simulink model "SSN_39busRT_Ctrl_4WT_19B"  (R2021a)
settings: Solver=ode3  StartTime=0.0  StopTime=10  FixedStep=Ts  MaxStep=1/60  RelTol=1e-2  AbsTol=1e-1
PreLoadFcn:
  | Ts=2.50e-6; ssn_ieee39_params; load('Pwf.mat');
InitFcn:
  | Ts=2.50e-6; ssn_ieee39_params; load('Pwf.mat');
values from neighbouring files (symbols this model uses):
  f = 50    [ssn_ieee39_params_ctrl.m]
  fNom = f    (= 60)    [ssn_ieee39_params_ctrl.m]
  ILR = 5.02    [ssn_ieee39_params_ctrl.m]
  IQMIN = 0.1    [ssn_ieee39_params_ctrl.m]
  ISCLIM = 1    [ssn_ieee39_params_ctrl.m]
  ITFpu = 1.10    (= 1.1)    [ssn_ieee39_params_ctrl.m]
  K = 1    [ssn_ieee39_params_ctrl.m]
  K1 = 1    [ssn_ieee39_params_ctrl.m]
  K2 = 2    [ssn_ieee39_params_ctrl.m]
  KCL = 1.04    [ssn_ieee39_params_ctrl.m]
  KFB = 0    [ssn_ieee39_params_ctrl.m]
  KFF = 1    [ssn_ieee39_params_ctrl.m]
  KFIX = 1    [ssn_ieee39_params_ctrl.m]
  KG = 1    [ssn_ieee39_params_ctrl.m]
  KIA = 59.91    [ssn_ieee39_params_ctrl.m]
  KIOEX = 0.0303    [ssn_ieee39_params_ctrl.m]
  KIUEX = 0.0303    [ssn_ieee39_params_ctrl.m]
  KIUOEX = 1    [ssn_ieee39_params_ctrl.m]
  KIUUEX = 1    [ssn_ieee39_params_ctrl.m]
  KLR = 22.47    [ssn_ieee39_params_ctrl.m]
  KM = 1    [ssn_ieee39_params_ctrl.m]
  KOEL = 0.24    [ssn_ieee39_params_ctrl.m]
  Kp = 1    [ssn_ieee39_params_ctrl.m]
  KPA = 30    [ssn_ieee39_params_ctrl.m]
  KPOEL = 1    [ssn_ieee39_params_ctrl.m]
  KPOEX = 0    [ssn_ieee39_params_ctrl.m]
  KPUEX = 0    [ssn_ieee39_params_ctrl.m]
  KSCALE = 0.319    [ssn_ieee39_params_ctrl.m]
  KUF = 0    [ssn_ieee39_params_ctrl.m]
  KUI = 0.001    [ssn_ieee39_params_ctrl.m]
  KUL = 0.24    [ssn_ieee39_params_ctrl.m]
  s = 10    [ssn_ieee39_params_ctrl.m]
  TA = 0.01    [ssn_ieee39_params_ctrl.m]
  Tadj = 0    [ssn_ieee39_params_ctrl.m]
  taps = [1 1 1.07 1.07 1.009 1.025 1 1.025 1.025 1.025]*1    [ssn_ieee39_params_ctrl.m]
  TF = 0.02    [ssn_ieee39_params_ctrl.m]
  TG = 0.024    [ssn_ieee39_params_ctrl.m]
  TINV = 0    [ssn_ieee39_params_ctrl.m]
  TIT = 0.1    [ssn_ieee39_params_ctrl.m]
  TL_10_11_len = 14    [ssn_ieee39_params_ctrl.m]
  TL_10_13_len = 14    [ssn_ieee39_params_ctrl.m]
  TL_13_14_len = 32    [ssn_ieee39_params_ctrl.m]
  TL_14_15_len = 70    [ssn_ieee39_params_ctrl.m]
  TL_15_16_len = 31.5    [ssn_ieee39_params_ctrl.m]
  TL_16_17_len = 26    [ssn_ieee39_params_ctrl.m]
  TL_16_19_len = 61    [ssn_ieee39_params_ctrl.m]
  TL_16_21_len = 46    [ssn_ieee39_params_ctrl.m]
  TL_16_24_len = 15    [ssn_ieee39_params_ctrl.m]
  TL_17_18_len = 26    [ssn_ieee39_params_ctrl.m]
  TL_17_27_len = 59    [ssn_ieee39_params_ctrl.m]
  TL_1_2_len = 134    [ssn_ieee39_params_ctrl.m]
  TL_1_39_len = 105    [ssn_ieee39_params_ctrl.m]
  TL_21_22_len = 47    [ssn_ieee39_params_ctrl.m]
  TL_22_23_len = 33    [ssn_ieee39_params_ctrl.m]
  TL_24_23_len = 88    [ssn_ieee39_params_ctrl.m]
  TL_25_26_len = 101    [ssn_ieee39_params_ctrl.m]
  TL_26_27_len = 46.5    [ssn_ieee39_params_ctrl.m]
  TL_26_28_len = 151    [ssn_ieee39_params_ctrl.m]
  TL_26_29_len = 200    [ssn_ieee39_params_ctrl.m]
  TL_28_29_len = 48    [ssn_ieee39_params_ctrl.m]
  TL_2_25_len = 28    [ssn_ieee39_params_ctrl.m]
  TL_2_2_len = 49    [ssn_ieee39_params_ctrl.m]
  TL_3_18_len = 42    [ssn_ieee39_params_ctrl.m]
  TL_3_4_len = 53    [ssn_ieee39_params_ctrl.m]
  TL_4_14_len = 33    [ssn_ieee39_params_ctrl.m]
  TL_4_5_len = 32.5    [ssn_ieee39_params_ctrl.m]
  TL_5_6_len = 14    [ssn_ieee39_params_ctrl.m]
  TL_5_8_len = 32    [ssn_ieee39_params_ctrl.m]
  TL_6_11_len = 26.5    [ssn_ieee39_params_ctrl.m]
  TL_6_7_len = 25.5    [ssn_ieee39_params_ctrl.m]
  TL_7_8_len = 15    [ssn_ieee39_params_ctrl.m]
  TL_8_9_len = 93    [ssn_ieee39_params_ctrl.m]
  TL_9_39_len = 136    [ssn_ieee39_params_ctrl.m]
  TOEL = 5.00    (= 5)    [ssn_ieee39_params_ctrl.m]
  TQREF = 0    [ssn_ieee39_params_ctrl.m]
  TQSCL = 0.012    [ssn_ieee39_params_ctrl.m]
  Ts_PMU = 1/1000    (= 0.001)    [ssn_ieee39_params_ctrl.m]
  TU1 = 0    [ssn_ieee39_params_ctrl.m]
  TU2 = 0    [ssn_ieee39_params_ctrl.m]
  TU3 = 0    [ssn_ieee39_params_ctrl.m]
  TU4 = 0    [ssn_ieee39_params_ctrl.m]
  TUL = 0    [ssn_ieee39_params_ctrl.m]
  TUP = 0.050    (= 0.05)    [ssn_ieee39_params_ctrl.m]
  TUQ = .005    (= 0.005)    [ssn_ieee39_params_ctrl.m]
  TUV = 0.2    [ssn_ieee39_params_ctrl.m]
  VAAMAX = VAMAX    (= 7.05)    [ssn_ieee39_params_ctrl.m]
  VAMAX = 7.05    [ssn_ieee39_params_ctrl.m]
  VAMIN = -6.11    [ssn_ieee39_params_ctrl.m]
  VBMAX = 999    [ssn_ieee39_params_ctrl.m]
  VF = 0    [ssn_ieee39_params_ctrl.m]
  VFB = 0    [ssn_ieee39_params_ctrl.m]
  VMMAX = 7.05    [ssn_ieee39_params_ctrl.m]
  VMMIN = -6.11    [ssn_ieee39_params_ctrl.m]
  VOELmax1 = 0.2353    [ssn_ieee39_params_ctrl.m]
  VOELmax2 = 0.0    (= 0)    [ssn_ieee39_params_ctrl.m]
  VOELmin1 = -0.24    [ssn_ieee39_params_ctrl.m]
  VOELmin2 = -1.0    (= -1)    [ssn_ieee39_params_ctrl.m]
  VRMAX = 7.05    [ssn_ieee39_params_ctrl.m]
  VRMIN = -6.11    [ssn_ieee39_params_ctrl.m]
  VSCLmax = 0.20    (= 0.2)    [ssn_ieee39_params_ctrl.m]
  VSCLmin = -0.10    (= -0.1)    [ssn_ieee39_params_ctrl.m]
  VUELmax1 = 1    [ssn_ieee39_params_ctrl.m]
  VUELmax2 = 1    [ssn_ieee39_params_ctrl.m]
  VUELmin1 = -1    [ssn_ieee39_params_ctrl.m]
  VUELmin2 = -1    [ssn_ieee39_params_ctrl.m]
  VUImax = 1    [ssn_ieee39_params_ctrl.m]
  VUImin = -1    [ssn_ieee39_params_ctrl.m]
undefined symbols (not defined in the file or in its folder): another_event_name, D1, Delta, DiscIntNeverNeededParam, find_system, MOV_segment9, my_event_name, powergui, Pw1, Pw2, Pw3, Pw4, vNomHV
libraries: powerlib_extras x162, spsThreePhaseVIMeasurementLib x55, spsCurrentMeasurementLib x52, simulink_extras x44, slpidlib x40, op_dpl_lib x36, spsST2AModel x20, spsThreePhaseParallelRLCLoadLib x20, spsThreePhaseTransformerTwoWindingsLib x17, spsControlledVoltageSourceLib x16, spsVoltageMeasurementLib x12, spsSynchronousMachinepuStandardLib x10
(part 18 of 19)

== system SSN_39busRT_Ctrl_4WT_19B/SM_master/4 WT/SS_windfarm3to4/Wind Farm (DFIG Type)/Wind Turbine Doubly-Fed Induction Generator (Average Model)1/Control System_average/Control/Rotor-side converter Control system/Priority Iqr ==
  Idqr* : Inport
  Cartesian to Polar : simulink_extras/Transformations/Cartesian to Polar
  Demux : Demux  Outputs=2
      settings: DisplayOption=none
  Irotor_max^2 : Constant
  Math Function : Math  Operator=square  SignedPower=on  SaturateOnIntegerOverflow=on
  Math Function1 : Math  Operator=sqrt  SignedPower=on  SaturateOnIntegerOverflow=on
  Mux : Mux  Inputs=2
  Mux1 : Mux  Inputs=2
  Product : Product  InputSameDT=on  SaturateOnIntegerOverflow=on  OutDataTypeStr=Inherit: Same as first input
  Rate Limiter : RateLimiter  RisingSlewLimit=current_slew_rate  FallingSlewLimit=-current_slew_rate
  Sign : Signum  ZeroCross=off
  Sum : Sum  Inputs=|+-  InputSameDT=on  SaturateOnIntegerOverflow=on  OutDataTypeStr=Inherit: Same as first input
  Switch : Switch  Threshold=1  SaturateOnIntegerOverflow=on  InputSameDT=on
  Terminator : Terminator
  Idqr_ref : Outport
  wires:
  Idqr*/1 -> Demux/1
  Rate Limiter/1 -> Idqr_ref/1
  Sign/1 -> Product/1
  Math Function1/1 -> Product/2
  Switch/1 -> Rate Limiter/1
  Mux1/1 -> Switch/1
  Sum/1 -> Math Function1/1
  Math Function/1 -> Sum/2
  Irotor_max^2/1 -> Sum/1
  Mux/1 -> Switch/3
  Cartesian to Polar/1 -> Switch/2
  Cartesian to Polar/2 -> Terminator/1
  Demux/1 -> Mux/1, Cartesian to Polar/1, Sign/1
  Demux/2 -> Mux/2, Cartesian to Polar/2, Math Function/1, Mux1/2
  Product/1 -> Mux1/1

== system SSN_39busRT_Ctrl_4WT_19B/SM_master/4 WT/SS_windfarm3to4/Wind Farm (DFIG Type)/Wind Turbine Doubly-Fed Induction Generator (Average Model)1/Control System_average/Control/Rotor-side converter Control system/Q Regulator ==
  Q_ref : Inport
  Q_B1 : Inport  Port=2
  Discrete PI Controller : powerlib_extras/Discrete  Control Blocks/Discrete PI Controller  Kp=Kp_Q  Ki=Ki_Q  Par_Limits=[1 -1]  Init=0  Ts=Ts_Control
  Rate Limiter : RateLimiter  RisingSlewLimit=current_slew_rate  FallingSlewLimit=-current_slew_rate
  "Rate Limiter " : RateLimiter  RisingSlewLimit=Q_slew_rate  FallingSlewLimit=-Q_slew_rate
  Sum : Sum  Inputs=|-+  InputSameDT=on  SaturateOnIntegerOverflow=on  OutDataTypeStr=Inherit: Same as first input
  Iqr* : Outport
  wires:
  "Rate Limiter "/1 -> Sum/1
  Rate Limiter/1 -> Iqr*/1
  Q_ref/1 -> "Rate Limiter "/1
  Sum/1 -> Discrete PI Controller/1
  Discrete PI Controller/1 -> Rate Limiter/1
  Q_B1/1 -> Sum/2

== system SSN_39busRT_Ctrl_4WT_19B/SM_master/4 WT/SS_windfarm3to4/Wind Farm (DFIG Type)/Wind Turbine Doubly-Fed Induction Generator (Average Model)1/Control System_average/Control/Rotor-side converter Control system/Torque control ==
  wr : Inport
  Idqr : Inport  Port=2
  Idqs : Inport  Port=3
  Idq_grid_conv : Inport  Port=4
  Freq : Inport  Port=5
  Vdqs : Inport  Port=6
  Torque reference : Subsystem
  Torque regulator : Subsystem
  Idr* : Outport
  wires:
  Idq_grid_conv/1 -> Torque reference/4(Idq_grid_conv)
  Idqr/1 -> Torque reference/3(Idqr)
  Idqs/1 -> Torque reference/2(Idqs), Torque regulator/3(Idqs)
  Torque reference/1(Torque_cmd) -> Torque regulator/1(Torque_cmd)
  wr/1 -> Torque reference/1(wr)
  Freq/1 -> Torque reference/5(Freq), Torque regulator/4(Freq)
  Torque regulator/1(Idr) -> Idr*/1
  Vdqs/1 -> Torque regulator/2(Vdqs)

== system SSN_39busRT_Ctrl_4WT_19B/SM_master/4 WT/SS_windfarm3to4/Wind Farm (DFIG Type)/Wind Turbine Doubly-Fed Induction Generator (Average Model)1/Control System_average/Control/Rotor-side converter Control system/Transformation abc --> dq  ==
  Theta : Inport
  Iabc_r : Inport  Port=2
  Iabc_s : Inport  Port=3
  Iabc_grid_conv : Inport  Port=4
  angle_rotor : Inport  Port=5
  # pairs of poles : Gain  Gain=p  SaturateOnIntegerOverflow=on  OutDataTypeStr=Inherit: Same as input  ParamDataTypeStr=Inherit: Same as input
  Constant4 : Constant  Value=2*pi
  Demux1 : Demux  Outputs=[2 1]
      settings: DisplayOption=none
  Demux2 : Demux  Outputs=[2 1]
      settings: DisplayOption=none
  Demux3 : Demux  Outputs=[2 1]
      settings: DisplayOption=none
  Math Function : Math  Operator=mod  SignedPower=on  SaturateOnIntegerOverflow=on
  Mux1 : Mux  Inputs=2
  Mux2 : Mux  Inputs=2
  Sum1 : Sum  Inputs=+-  InputSameDT=on  SaturateOnIntegerOverflow=on  OutDataTypeStr=Inherit: Same as first input
  Terminator1 : Terminator
  Terminator2 : Terminator
  Terminator3 : Terminator
  Trigonometric Function1 : Trigonometry
  Trigonometric Function2 : Trigonometry
  Trigonometric Function3 : Trigonometry  Operator=cos
  Trigonometric Function4 : Trigonometry  Operator=cos
  abc_to_dq0 : powerlib_extras/Measurements/abc_to_dq0 Transformation
      settings: SourceProductBaseCode=PS
  "abc_to_dq0 " : powerlib_extras/Measurements/abc_to_dq0 Transformation
      settings: SourceProductBaseCode=PS
  "abc_to_dq0  " : powerlib_extras/Measurements/abc_to_dq0 Transformation
      settings: SourceProductBaseCode=PS
  Idq_r : Outport
  Idq_s : Outport  Port=2
  Idq_gc : Outport  Port=3
  r_angle_transformation : Outport  Port=4
  wires:
  "abc_to_dq0 "/1 -> Demux1/1
  Trigonometric Function2/1 -> Mux1/1
  Trigonometric Function3/1 -> Mux1/2
  Mux1/1 -> "abc_to_dq0  "/2
  Demux1/2 -> Terminator1/1
  Demux1/1 -> Idq_s/1
  Iabc_s/1 -> "abc_to_dq0 "/1
  "abc_to_dq0  "/1 -> Demux2/1
  Demux2/2 -> Terminator2/1
  Demux2/1 -> Idq_r/1
  Iabc_r/1 -> "abc_to_dq0  "/1
  angle_rotor/1 -> # pairs of poles/1
  Theta/1 -> Sum1/1, Trigonometric Function4/1, Trigonometric Function1/1
  Sum1/1 -> r_angle_transformation/1, Trigonometric Function3/1, Trigonometric Function2/1
  Trigonometric Function1/1 -> Mux2/1
  Trigonometric Function4/1 -> Mux2/2
  Mux2/1 -> "abc_to_dq0 "/2, abc_to_dq0/2
  abc_to_dq0/1 -> Demux3/1
  Demux3/2 -> Terminator3/1
  Demux3/1 -> Idq_gc/1
  Iabc_grid_conv/1 -> abc_to_dq0/1
  Constant4/1 -> Math Function/2
  # pairs of poles/1 -> Math Function/1
  Math Function/1 -> Sum1/2

== system SSN_39busRT_Ctrl_4WT_19B/SM_master/4 WT/SS_windfarm3to4/Wind Farm (DFIG Type)/Wind Turbine Doubly-Fed Induction Generator (Average Model)1/Control System_average/Control/Rotor-side converter Control system/dq --> abc ==
  note: Required value for modulation index "m" to obtain 1 pu generated voltage by the converter:
  note: m = Vnom_r * 2*sqrt(2/3) / Vdc
  note: Where Vnom_r = RMS ph-ph nominal voltage
  Vdq* : Inport
  Vdc : Inport  Port=2
  Angle : Inport  Port=3
  0-1 : Saturate  UpperLimit=1  LowerLimit=0
  Avoid division by zero : Saturate  UpperLimit=1e6  LowerLimit=1e-6
  Cartesian to Polar : simulink_extras/Transformations/Cartesian to Polar
  Demux1 : Demux  Outputs=2
      settings: DisplayOption=none
  K : Constant  Value=Vnom*2*sqrt(2/3)
  Mux1 : Mux  Inputs=3
  Mux2 : Mux  Inputs=2
  Polar to Cartesian : simulink_extras/Transformations/Polar to Cartesian
      settings: SourceProductBaseCode=SL
  Product2 : Product  Inputs=**/  InputSameDT=on  SaturateOnIntegerOverflow=on  OutDataTypeStr=Inherit: Same as first input
  Trigonometric Function2 : Trigonometry
  Trigonometric Function3 : Trigonometry  Operator=cos
  V0 : Constant  Value=0
  dq0_to_abc Transformation : powerlib_extras/Measurements/dq0_to_abc Transformation
      settings: SourceProductBaseCode=PS
  Uctrl_rotor_conv : Outport
  wires:
  Mux2/1 -> dq0_to_abc Transformation/2
  Trigonometric Function2/1 -> Mux2/1
  Trigonometric Function3/1 -> Mux2/2
  Angle/1 -> Trigonometric Function3/1, Trigonometric Function2/1
  dq0_to_abc Transformation/1 -> Uctrl_rotor_conv/1
  V0/1 -> Mux1/3
  Polar to Cartesian/1 -> Mux1/1
  Polar to Cartesian/2 -> Mux1/2
  0-1/1 -> Polar to Cartesian/1
  Product2/1 -> 0-1/1  "m"
  Vdc/1 -> Avoid division by zero/1
  K/1 -> Product2/2
  Avoid division by zero/1 -> Product2/3
  Demux1/1 -> Cartesian to Polar/1
  Demux1/2 -> Cartesian to Polar/2
  Cartesian to Polar/1 -> Product2/1
  Cartesian to Polar/2 -> Polar to Cartesian/2
  Vdq*/1 -> Demux1/1
  Mux1/1 -> dq0_to_abc Transformation/1  "Vdq0"

== system SSN_39busRT_Ctrl_4WT_19B/SM_master/4 WT/SS_windfarm3to4/Wind Farm (DFIG Type)2/Wind Turbine Doubly-Fed Induction Generator (Average Model)1/Control System_average/Control/Grid-side converter Control system/Current regulator ==
  Vdqs : Inport
  Idq : Inport  Port=2
  Freq : Inport  Port=3
  Idq_ref : Inport  Port=4
  Constant1 : Constant  Value=L_RL
  Constant2 : Constant  Value=L_RL
  Constant3 : Constant  Value=R_RL
  Constant4 : Constant  Value=R_RL
  Demux{,1..3} (4 alike) : Demux  Outputs=2
      settings: DisplayOption=none
  Discrete PI Controller : powerlib_extras/Discrete  Control Blocks/Discrete PI Controller  Kp=Kpi_grid_side_cur_reg(1)  Ki=Kpi_grid_side_cur_reg(2)  Par_Limits=[1.1 -1.1]  Init=0  Ts=Ts_Control
  Divide3 : Product  Inputs=*/
  Fnom : Constant  Value=Fnom
  Mux : Mux  Inputs=2
  Mux1 : Mux  Inputs=2
  Product : Product  Inputs=3  InputSameDT=on  SaturateOnIntegerOverflow=on  OutDataTypeStr=Inherit: Same as first input
  Product1 : Product  Inputs=3  InputSameDT=on  SaturateOnIntegerOverflow=on  OutDataTypeStr=Inherit: Same as first input
  Product2 : Product  InputSameDT=on  SaturateOnIntegerOverflow=on  OutDataTypeStr=Inherit: Same as first input
  Product3 : Product  InputSameDT=on  SaturateOnIntegerOverflow=on  OutDataTypeStr=Inherit: Same as first input
  Sum1 : Sum  Inputs=|+-  InputSameDT=on  SaturateOnIntegerOverflow=on  OutDataTypeStr=Inherit: Same as first input
  Sum2 : Sum  Inputs=-+|  InputSameDT=on  SaturateOnIntegerOverflow=on  OutDataTypeStr=Inherit: Same as first input
  Sum3 : Sum  Inputs=||++-  InputSameDT=on  SaturateOnIntegerOverflow=on  OutDataTypeStr=Inherit: Same as first input
  Sum4 : Sum  Inputs=|+-  InputSameDT=on  SaturateOnIntegerOverflow=on  OutDataTypeStr=Inherit: Same as first input
  Sum5 : Sum  Inputs=|--+  InputSameDT=on  SaturateOnIntegerOverflow=on  OutDataTypeStr=Inherit: Same as first input
  Sum6 : Sum  Inputs=|-+  InputSameDT=on  SaturateOnIntegerOverflow=on  OutDataTypeStr=Inherit: Same as first input
  Vdq* : Outport
  wires:
  [idr] -> Product1/1
  [iqr] -> Product3/1
  [idr] -> Product2/2
  [iqr] -> Product/3
  [w_pu] -> Product/2
  [w_pu] -> Product1/3
  Divide3/1 -> [w_pu]
  Fnom/1 -> Divide3/2
  Freq/1 -> Divide3/1
  Sum2/1 -> Mux1/2
  Sum4/1 -> Mux1/1
  Sum3/1 -> Sum1/1
  Sum5/1 -> Sum6/2
  Product3/1 -> Sum5/1
  Product2/1 -> Sum3/3
  Demux2/2 -> Sum5/3  "Vq"
  Product1/1 -> Sum5/2
  Constant4/1 -> Product3/2
  Constant3/1 -> Product2/1
  Product/1 -> Sum3/2
  Demux3/2 -> Sum6/1  "vq'"
  Mux/1 -> Vdq*/1
  Sum1/1 -> Mux/1
  Sum6/1 -> Mux/2
  Idq/1 -> Demux/1
  Demux/1 -> Sum4/2  "Id"
  Demux/2 -> Sum2/1  "Iq"
  Demux1/1 -> [idr], Sum4/1  "Id_ref"
  Idq_ref/1 -> Demux1/1
  Demux1/2 -> [iqr], Sum2/2  "Iq_ref"
  Vdqs/1 -> Demux2/1
  Constant1/1 -> Product/1
  Demux2/1 -> Sum3/1  "Vd"
  Mux1/1 -> Discrete PI Controller/1
  Discrete PI Controller/1 -> Demux3/1
  Demux3/1 -> Sum1/2  "vd'"
  Constant2/1 -> Product1/2

== system SSN_39busRT_Ctrl_4WT_19B/SM_master/4 WT/SS_windfarm3to4/Wind Farm (DFIG Type)2/Wind Turbine Doubly-Fed Induction Generator (Average Model)1/Control System_average/Control/Grid-side converter Control system/DC bus voltage Regulator ==
  Vdc_ref : Inport
  Vdc : Inport  Port=2
  Discrete PI Controller : powerlib_extras/Discrete  Control Blocks/Discrete PI Controller  Kp=Kpi_dc_reg(1)  Ki=Kpi_dc_reg(2)  Par_Limits=[1 -1]*Imax_grid_conv  Init=0  Ts=Ts_Control
  Rate Limiter : RateLimiter  RisingSlewLimit=current_slew_rate  FallingSlewLimit=-current_slew_rate
  Sum7 : Sum  Inputs=|+-  InputSameDT=on  SaturateOnIntegerOverflow=on  OutDataTypeStr=Inherit: Same as first input
  Id_ref : Outport
  wires:
  Rate Limiter/1 -> Id_ref/1
  Vdc/1 -> Sum7/2
  Discrete PI Controller/1 -> Rate Limiter/1
  Vdc_ref/1 -> Sum7/1
  Sum7/1 -> Discrete PI Controller/1

== system SSN_39busRT_Ctrl_4WT_19B/SM_master/4 WT/SS_windfarm3to4/Wind Farm (DFIG Type)2/Wind Turbine Doubly-Fed Induction Generator (Average Model)1/Control System_average/Control/Grid-side converter Control system/Idq references ==
  Id*Iq* : Inport
  Cartesian to Polar : simulink_extras/Transformations/Cartesian to Polar
  Demux : Demux  Outputs=2
      settings: DisplayOption=none
  Igrid_conv_max^2 : Constant  Value=Imax_grid_conv^2
  Math Function : Math  Operator=square  SignedPower=on  SaturateOnIntegerOverflow=on
  Math Function1 : Math  Operator=sqrt  SignedPower=on  SaturateOnIntegerOverflow=on
  Mux : Mux  Inputs=2
  Mux1 : Mux  Inputs=2
  Product : Product  InputSameDT=on  SaturateOnIntegerOverflow=on  OutDataTypeStr=Inherit: Same as first input
  Rate Limiter : RateLimiter  RisingSlewLimit=current_slew_rate  FallingSlewLimit=-current_slew_rate
  Sign : Signum  ZeroCross=off
  Sum : Sum  Inputs=|+-  InputSameDT=on  SaturateOnIntegerOverflow=on  OutDataTypeStr=Inherit: Same as first input
  Switch : Switch  Threshold=Imax_grid_conv  SaturateOnIntegerOverflow=on  InputSameDT=on
  Terminator : Terminator
  Idq_ref : Outport
  wires:
  Product/1 -> Mux1/2
  Rate Limiter/1 -> Idq_ref/1
  Demux/2 -> Cartesian to Polar/2, Mux/2, Sign/1
  Demux/1 -> Mux1/1, Math Function/1, Cartesian to Polar/1, Mux/1
  Cartesian to Polar/2 -> Terminator/1
  Cartesian to Polar/1 -> Switch/2
  Mux/1 -> Switch/3
  Igrid_conv_max^2/1 -> Sum/1
  Math Function/1 -> Sum/2
  Sum/1 -> Math Function1/1
  Mux1/1 -> Switch/1
  Switch/1 -> Rate Limiter/1
  Math Function1/1 -> Product/2  "Iq"
  Sign/1 -> Product/1
  Id*Iq*/1 -> Demux/1

== system SSN_39busRT_Ctrl_4WT_19B/SM_master/4 WT/SS_windfarm3to4/Wind Farm (DFIG Type)2/Wind Turbine Doubly-Fed Induction Generator (Average Model)1/Control System_average/Control/Grid-side converter Control system/Subsystem1 ==
  note: Where Vnom = RMS ph-ph nominal voltage
  note: m = Vnom * 2*sqrt(2/3) / Vdc
  note: Required value for modulation index "m" to obtain 1 pu generated voltage by the converter:
  Theta : Inport
  Vdq* : Inport  Port=2
  Vdc : Inport  Port=3
  0-1 : Saturate  UpperLimit=1  LowerLimit=0
  Avoid division by zero : Saturate  UpperLimit=1e6  LowerLimit=1e-6
  Cartesian to Polar1 : simulink_extras/Transformations/Cartesian to Polar
  Demux1 : Demux  Outputs=2
      settings: DisplayOption=none
  K : Constant  Value=Vnom*2*sqrt(2/3)
  Mux : Mux  Inputs=3
  Mux1 : Mux  Inputs=2
  Polar to Cartesian : simulink_extras/Transformations/Polar to Cartesian
      settings: SourceProductBaseCode=SL
  Product1 : Product  Inputs=**/  InputSameDT=on  SaturateOnIntegerOverflow=on  OutDataTypeStr=Inherit: Same as first input
  Trigonometric Function2 : Trigonometry
  Trigonometric Function3 : Trigonometry  Operator=cos
  V0 : Constant  Value=0
  dq0_to_abc Transformation : powerlib_extras/Measurements/dq0_to_abc Transformation
      settings: SourceProductBaseCode=PS
  Uctrl_grid_conv : Outport
  wires:
  Cartesian to Polar1/2 -> Polar to Cartesian/2
  Cartesian to Polar1/1 -> Product1/1
  Demux1/2 -> Cartesian to Polar1/2
  Demux1/1 -> Cartesian to Polar1/1
  Theta/1 -> Trigonometric Function3/1, Trigonometric Function2/1
  Vdq*/1 -> Demux1/1
  Avoid division by zero/1 -> Product1/3
  K/1 -> Product1/2
  Vdc/1 -> Avoid division by zero/1
  Product1/1 -> 0-1/1  "m"
  0-1/1 -> Polar to Cartesian/1
  Mux/1 -> dq0_to_abc Transformation/1  "Vdq0"
  Polar to Cartesian/2 -> Mux/2
  Polar to Cartesian/1 -> Mux/1
  dq0_to_abc Transformation/1 -> Uctrl_grid_conv/1
  V0/1 -> Mux/3
  Trigonometric Function3/1 -> Mux1/2
  Trigonometric Function2/1 -> Mux1/1
  Mux1/1 -> dq0_to_abc Transformation/2

== system SSN_39busRT_Ctrl_4WT_19B/SM_master/4 WT/SS_windfarm3to4/Wind Farm (DFIG Type)2/Wind Turbine Doubly-Fed Induction Generator (Average Model)1/Control System_average/Control/Grid-side converter Control system/Transformation abc --> dq ==
  Theta : Inport
  Vabc : Inport  Port=2
  Iabc : Inport  Port=3
  Demux1 : Demux  Outputs=[2 1]
      settings: DisplayOption=none
  Demux3 : Demux  Outputs=[2 1]
      settings: DisplayOption=none
  Mux1 : Mux  Inputs=2
  Terminator1 : Terminator
  Terminator3 : Terminator
  Trigonometric Function2 : Trigonometry
  Trigonometric Function3 : Trigonometry  Operator=cos
  abc_to_dq0 : powerlib_extras/Measurements/abc_to_dq0 Transformation
      settings: SourceProductBaseCode=PS
  "abc_to_dq0  " : powerlib_extras/Measurements/abc_to_dq0 Transformation
      settings: SourceProductBaseCode=PS
  Vdq : Outport
  Idq : Outport  Port=2
  wires:
  Iabc/1 -> "abc_to_dq0  "/1
  Demux1/1 -> Idq/1
  Demux1/2 -> Terminator1/1
  Demux3/1 -> Vdq/1
  Demux3/2 -> Terminator3/1
  Mux1/1 -> abc_to_dq0/2, "abc_to_dq0  "/2
  Trigonometric Function3/1 -> Mux1/2
  Trigonometric Function2/1 -> Mux1/1
  "abc_to_dq0  "/1 -> Demux1/1
  Vabc/1 -> abc_to_dq0/1
  abc_to_dq0/1 -> Demux3/1
  Theta/1 -> Trigonometric Function2/1, Trigonometric Function3/1

== system SSN_39busRT_Ctrl_4WT_19B/SM_master/4 WT/SS_windfarm3to4/Wind Farm (DFIG Type)2/Wind Turbine Doubly-Fed Induction Generator (Average Model)1/Control System_average/Control/Rotor-side converter Control system/Current Regulator ==
  note: Current regulator
  Idqr_ref : Inport
  Idq_r : Inport  Port=2
  Idq_s : Inport  Port=3
  wr : Inport  Port=4
  Freq : Inport  Port=5
  Demux{,1..3} (4 alike) : Demux  Outputs=2
      settings: DisplayOption=none
  Discrete PI Controller : powerlib_extras/Discrete  Control Blocks/Discrete PI Controller  Kp=Kpi_rotor_side_cur_reg(1)  Ki=Kpi_rotor_side_cur_reg(2)  Par_Limits=[0.1 -0.1]  Init=0  Ts=Ts_Control
  Divide3 : Product  Inputs=*/
  Fnom : Constant  Value=Fnom
  Llr+Lm1 : Constant  Value=Llr+Lm
  Llr+Lm2 : Constant  Value=Llr+Lm
  Lm1 : Constant  Value=Lm
  Lm2 : Constant  Value=Lm
  Lm3 : Constant  Value=Rr
  Lm4 : Constant  Value=Rr
  Mux1 : Mux  Inputs=2
  Mux2 : Mux  Inputs=2
  Product{1..4} (4 alike) : Product  Inputs=3  SaturateOnIntegerOverflow=on  OutDataTypeStr=Inherit: Same as first input
  Product5 : Product  SaturateOnIntegerOverflow=on  OutDataTypeStr=Inherit: Same as first input
  Product6 : Product  SaturateOnIntegerOverflow=on  OutDataTypeStr=Inherit: Same as first input
  Sum1 : Sum  Inputs=|+-  InputSameDT=on  SaturateOnIntegerOverflow=on  OutDataTypeStr=Inherit: Same as first input
  Sum2 : Sum  Inputs=+--  InputSameDT=on  SaturateOnIntegerOverflow=on  OutDataTypeStr=Inherit: Same as first input
  Sum3 : Sum  Inputs=-+|  InputSameDT=on  SaturateOnIntegerOverflow=on  OutDataTypeStr=Inherit: Same as first input
  Sum4 : Sum  Inputs=|+-  InputSameDT=on  SaturateOnIntegerOverflow=on  OutDataTypeStr=Inherit: Same as first input
  Sum5 : Sum  InputSameDT=on  SaturateOnIntegerOverflow=on  OutDataTypeStr=Inherit: Same as first input
  Sum6 : Sum  Inputs=+++  InputSameDT=on  SaturateOnIntegerOverflow=on  OutDataTypeStr=Inherit: Same as first input
  Sum7 : Sum  InputSameDT=on  SaturateOnIntegerOverflow=on  OutDataTypeStr=Inherit: Same as first input
  Vdq* : Outport
  wires:
  Sum6/1 -> Sum7/2
  Demux3/2 -> Sum7/1  "vq'"
  Demux3/1 -> Sum5/2  "vd'"
  Fnom/1 -> Divide3/2
  Freq/1 -> Divide3/1
  Sum5/1 -> Mux2/1
  Sum2/1 -> Sum5/1
  Product5/1 -> Sum6/3
  Product3/1 -> Sum6/1
  Product2/1 -> Sum2/2
  Product6/1 -> Sum2/1
  [idr] -> Product3/3
  [iqr] -> Product5/2
  [iqr] -> Product2/3
  [idr] -> Product6/2
  Demux/2 -> [iqr], Sum3/1  "Iqr"
  Demux/1 -> [idr], Sum4/2  "Idr"
  Idqr_ref/1 -> Demux1/1
  Discrete PI Controller/1 -> Demux3/1
  Product1/1 -> Sum2/3
  Lm4/1 -> Product6/1
  Lm3/1 -> Product5/1
  Product4/1 -> Sum6/2
  Mux2/1 -> Vdq*/1
  Sum7/1 -> Mux2/2
  Lm2/1 -> Product4/2
  [w_wr] -> Product4/1
  [ids] -> Product4/3
  Llr+Lm2/1 -> Product3/2
  [w_wr] -> Product3/1
  Lm1/1 -> Product1/2
  [w_wr] -> Product1/1
  [iqs] -> Product1/3
  Llr+Lm1/1 -> Product2/2
  [w_wr] -> Product2/1
  Sum1/1 -> [w_wr]  "w-wr"
  Demux2/2 -> [iqs]
  Demux2/1 -> [ids]
  wr/1 -> Sum1/2
  Divide3/1 -> Sum1/1
  Idq_s/1 -> Demux2/1
  Mux1/1 -> Discrete PI Controller/1
  Demux1/2 -> Sum3/2  "Iqr*"
  Demux1/1 -> Sum4/1  "Idr*"
  Sum3/1 -> Mux1/2
  Sum4/1 -> Mux1/1
  Idq_r/1 -> Demux/1

== system SSN_39busRT_Ctrl_4WT_19B/SM_master/4 WT/SS_windfarm3to4/Wind Farm (DFIG Type)2/Wind Turbine Doubly-Fed Induction Generator (Average Model)1/Control System_average/Control/Rotor-side converter Control system/Priority Iqr ==
  Idqr* : Inport
  Cartesian to Polar : simulink_extras/Transformations/Cartesian to Polar
  Demux : Demux  Outputs=2
      settings: DisplayOption=none
  Irotor_max^2 : Constant
  Math Function : Math  Operator=square  SignedPower=on  SaturateOnIntegerOverflow=on
  Math Function1 : Math  Operator=sqrt  SignedPower=on  SaturateOnIntegerOverflow=on
  Mux : Mux  Inputs=2
  Mux1 : Mux  Inputs=2
  Product : Product  InputSameDT=on  SaturateOnIntegerOverflow=on  OutDataTypeStr=Inherit: Same as first input
  Rate Limiter : RateLimiter  RisingSlewLimit=current_slew_rate  FallingSlewLimit=-current_slew_rate
  Sign : Signum  ZeroCross=off
  Sum : Sum  Inputs=|+-  InputSameDT=on  SaturateOnIntegerOverflow=on  OutDataTypeStr=Inherit: Same as first input
  Switch : Switch  Threshold=1  SaturateOnIntegerOverflow=on  InputSameDT=on
  Terminator : Terminator
  Idqr_ref : Outport
  wires:
  Product/1 -> Mux1/1
  Demux/2 -> Mux1/2, Math Function/1, Cartesian to Polar/2, Mux/2
  Demux/1 -> Sign/1, Cartesian to Polar/1, Mux/1
  Cartesian to Polar/2 -> Terminator/1
  Cartesian to Polar/1 -> Switch/2
  Mux/1 -> Switch/3
  Irotor_max^2/1 -> Sum/1
  Math Function/1 -> Sum/2
  Sum/1 -> Math Function1/1
  Mux1/1 -> Switch/1
  Switch/1 -> Rate Limiter/1
  Math Function1/1 -> Product/2
  Sign/1 -> Product/1
  Rate Limiter/1 -> Idqr_ref/1
  Idqr*/1 -> Demux/1

== system SSN_39busRT_Ctrl_4WT_19B/SM_master/4 WT/SS_windfarm3to4/Wind Farm (DFIG Type)2/Wind Turbine Doubly-Fed Induction Generator (Average Model)1/Control System_average/Control/Rotor-side converter Control system/Q Regulator ==
  Q_ref : Inport
  Q_B1 : Inport  Port=2
  Discrete PI Controller : powerlib_extras/Discrete  Control Blocks/Discrete PI Controller  Kp=Kp_Q  Ki=Ki_Q  Par_Limits=[1 -1]  Init=0  Ts=Ts_Control
  Rate Limiter : RateLimiter  RisingSlewLimit=current_slew_rate  FallingSlewLimit=-current_slew_rate
  "Rate Limiter " : RateLimiter  RisingSlewLimit=Q_slew_rate  FallingSlewLimit=-Q_slew_rate
  Sum : Sum  Inputs=|-+  InputSameDT=on  SaturateOnIntegerOverflow=on  OutDataTypeStr=Inherit: Same as first input
  Iqr* : Outport
  wires:
  Q_B1/1 -> Sum/2
  Discrete PI Controller/1 -> Rate Limiter/1
  Sum/1 -> Discrete PI Controller/1
  Q_ref/1 -> "Rate Limiter "/1
  Rate Limiter/1 -> Iqr*/1
  "Rate Limiter "/1 -> Sum/1

== system SSN_39busRT_Ctrl_4WT_19B/SM_master/4 WT/SS_windfarm3to4/Wind Farm (DFIG Type)2/Wind Turbine Doubly-Fed Induction Generator (Average Model)1/Control System_average/Control/Rotor-side converter Control system/Torque control ==
  wr : Inport
  Idqr : Inport  Port=2
  Idqs : Inport  Port=3
  Idq_grid_conv : Inport  Port=4
  Freq : Inport  Port=5
  Vdqs : Inport  Port=6
  Torque reference : Subsystem
  Torque regulator : Subsystem
  Idr* : Outport
  wires:
  Vdqs/1 -> Torque regulator/2(Vdqs)
  Torque regulator/1(Idr) -> Idr*/1
  Freq/1 -> Torque regulator/4(Freq), Torque reference/5(Freq)
  wr/1 -> Torque reference/1(wr)
  Torque reference/1(Torque_cmd) -> Torque regulator/1(Torque_cmd)
  Idqs/1 -> Torque regulator/3(Idqs), Torque reference/2(Idqs)
  Idqr/1 -> Torque reference/3(Idqr)
  Idq_grid_conv/1 -> Torque reference/4(Idq_grid_conv)

== system SSN_39busRT_Ctrl_4WT_19B/SM_master/4 WT/SS_windfarm3to4/Wind Farm (DFIG Type)2/Wind Turbine Doubly-Fed Induction Generator (Average Model)1/Control System_average/Control/Rotor-side converter Control system/Transformation abc --> dq  ==
  Theta : Inport
  Iabc_r : Inport  Port=2
  Iabc_s : Inport  Port=3
  Iabc_grid_conv : Inport  Port=4
  angle_rotor : Inport  Port=5
  # pairs of poles : Gain  Gain=p  SaturateOnIntegerOverflow=on  OutDataTypeStr=Inherit: Same as input  ParamDataTypeStr=Inherit: Same as input
  Constant4 : Constant  Value=2*pi
  Demux1 : Demux  Outputs=[2 1]
      settings: DisplayOption=none
  Demux2 : Demux  Outputs=[2 1]
      settings: DisplayOption=none
  Demux3 : Demux  Outputs=[2 1]
      settings: DisplayOption=none
  Math Function : Math  Operator=mod  SignedPower=on  SaturateOnIntegerOverflow=on
  Mux1 : Mux  Inputs=2
  Mux2 : Mux  Inputs=2
  Sum1 : Sum  Inputs=+-  InputSameDT=on  SaturateOnIntegerOverflow=on  OutDataTypeStr=Inherit: Same as first input
  Terminator1 : Terminator
  Terminator2 : Terminator
  Terminator3 : Terminator
  Trigonometric Function1 : Trigonometry
  Trigonometric Function2 : Trigonometry
  Trigonometric Function3 : Trigonometry  Operator=cos
  Trigonometric Function4 : Trigonometry  Operator=cos
  abc_to_dq0 : powerlib_extras/Measurements/abc_to_dq0 Transformation
      settings: SourceProductBaseCode=PS
  "abc_to_dq0 " : powerlib_extras/Measurements/abc_to_dq0 Transformation
      settings: SourceProductBaseCode=PS
  "abc_to_dq0  " : powerlib_extras/Measurements/abc_to_dq0 Transformation
      settings: SourceProductBaseCode=PS
  Idq_r : Outport
  Idq_s : Outport  Port=2
  Idq_gc : Outport  Port=3
  r_angle_transformation : Outport  Port=4
  wires:
  Math Function/1 -> Sum1/2
  # pairs of poles/1 -> Math Function/1
  Constant4/1 -> Math Function/2
  Iabc_grid_conv/1 -> abc_to_dq0/1
  Demux3/1 -> Idq_gc/1
  Demux3/2 -> Terminator3/1
  abc_to_dq0/1 -> Demux3/1
  Mux2/1 -> abc_to_dq0/2, "abc_to_dq0 "/2
  Trigonometric Function4/1 -> Mux2/2
  Trigonometric Function1/1 -> Mux2/1
  Sum1/1 -> Trigonometric Function2/1, Trigonometric Function3/1, r_angle_transformation/1
  Theta/1 -> Trigonometric Function1/1, Trigonometric Function4/1, Sum1/1
  angle_rotor/1 -> # pairs of poles/1
  Iabc_r/1 -> "abc_to_dq0  "/1
  Demux2/1 -> Idq_r/1
  Demux2/2 -> Terminator2/1
  "abc_to_dq0  "/1 -> Demux2/1
  Iabc_s/1 -> "abc_to_dq0 "/1
  Demux1/1 -> Idq_s/1
  Demux1/2 -> Terminator1/1
  Mux1/1 -> "abc_to_dq0  "/2
  Trigonometric Function3/1 -> Mux1/2
  Trigonometric Function2/1 -> Mux1/1
  "abc_to_dq0 "/1 -> Demux1/1

== system SSN_39busRT_Ctrl_4WT_19B/SM_master/4 WT/SS_windfarm3to4/Wind Farm (DFIG Type)2/Wind Turbine Doubly-Fed Induction Generator (Average Model)1/Control System_average/Control/Rotor-side converter Control system/dq --> abc ==
  note: Where Vnom_r = RMS ph-ph nominal voltage
  note: m = Vnom_r * 2*sqrt(2/3) / Vdc
  note: Required value for modulation index "m" to obtain 1 pu generated voltage by the converter:
  Vdq* : Inport
  Vdc : Inport  Port=2
  Angle : Inport  Port=3
  0-1 : Saturate  UpperLimit=1  LowerLimit=0
  Avoid division by zero : Saturate  UpperLimit=1e6  LowerLimit=1e-6
  Cartesian to Polar : simulink_extras/Transformations/Cartesian to Polar
  Demux1 : Demux  Outputs=2
      settings: DisplayOption=none
  K : Constant  Value=Vnom*2*sqrt(2/3)
  Mux1 : Mux  Inputs=3
  Mux2 : Mux  Inputs=2
  Polar to Cartesian : simulink_extras/Transformations/Polar to Cartesian
      settings: SourceProductBaseCode=SL
  Product2 : Product  Inputs=**/  InputSameDT=on  SaturateOnIntegerOverflow=on  OutDataTypeStr=Inherit: Same as first input
  Trigonometric Function2 : Trigonometry
  Trigonometric Function3 : Trigonometry  Operator=cos
  V0 : Constant  Value=0
  dq0_to_abc Transformation : powerlib_extras/Measurements/dq0_to_abc Transformation
      settings: SourceProductBaseCode=PS
  Uctrl_rotor_conv : Outport
  wires:
  Mux1/1 -> dq0_to_abc Transformation/1  "Vdq0"
  Vdq*/1 -> Demux1/1
  Cartesian to Polar/2 -> Polar to Cartesian/2
  Cartesian to Polar/1 -> Product2/1
  Demux1/2 -> Cartesian to Polar/2
  Demux1/1 -> Cartesian to Polar/1
  Avoid division by zero/1 -> Product2/3
  K/1 -> Product2/2
  Vdc/1 -> Avoid division by zero/1
  Product2/1 -> 0-1/1  "m"
  0-1/1 -> Polar to Cartesian/1
  Polar to Cartesian/2 -> Mux1/2
  Polar to Cartesian/1 -> Mux1/1
  V0/1 -> Mux1/3
  dq0_to_abc Transformation/1 -> Uctrl_rotor_conv/1
  Angle/1 -> Trigonometric Function2/1, Trigonometric Function3/1
  Trigonometric Function3/1 -> Mux2/2
  Trigonometric Function2/1 -> Mux2/1
  Mux2/1 -> dq0_to_abc Transformation/2

== system SSN_39busRT_Ctrl_4WT_19B/SM_master/4 WT/SS_windfarm1to2/Wind Farm (DFIG Type)/Wind Turbine Doubly-Fed Induction Generator (Average Model)1/Control System_average/Control/Rotor-side converter Control system/Torque control/Torque reference ==
  wr : Inport
  Idqs : Inport  Port=2
  Idqr : Inport  Port=3
  Idq_grid_conv : Inport  Port=4
  Freq : Inport  Port=5
  0-1 : Saturate  UpperLimit=1  LowerLimit=0
  0-inf : Saturate  UpperLimit=inf  LowerLimit=0
  "0-inf " : Saturate  UpperLimit=inf  LowerLimit=0
  0-power_C : Saturate  UpperLimit=power_C  LowerLimit=0
  1e-6-inf : Saturate  UpperLimit=inf  LowerLimit=1e-6
  Constant : Constant  Value=speed_C
  Constant1 : Constant  Value=speed_A
  "Gain " : Gain  Gain=power_C  SaturateOnIntegerOverflow=on  OutDataTypeStr=Inherit: Same as input  ParamDataTypeStr=Inherit: Same as input
  Looses : Subsystem
  Product1 : Product  SaturateOnIntegerOverflow=on  OutDataTypeStr=Inherit: Same as first input
  Product2 : Product  Inputs=*/  SaturateOnIntegerOverflow=on  OutDataTypeStr=Inherit: Same as first input
  Product3 : Product  SaturateOnIntegerOverflow=on  OutDataTypeStr=Inherit: Same as first input
  Slope_B_A : Subsystem
  Slope_D_C : Subsystem
  Sum2 : Sum  Inputs=|-+  SaturateOnIntegerOverflow=on
  Sum3 : Sum  Inputs=|++  SaturateOnIntegerOverflow=on
  Sum4 : Sum  Inputs=|+-  SaturateOnIntegerOverflow=on
  Sum5 : Sum  Inputs=|+-  SaturateOnIntegerOverflow=on
  Switch : Switch  Threshold=speed_B  SaturateOnIntegerOverflow=on
  "pu->pu " : Gain  Gain=1/speed_C  SaturateOnIntegerOverflow=on  OutDataTypeStr=Inherit: Same as input  ParamDataTypeStr=Inherit: Same as input
  "pu->pu  " : Gain  Gain=Pmec/Pnom  SaturateOnIntegerOverflow=on  OutDataTypeStr=Inherit: Same as input  ParamDataTypeStr=Inherit: Same as input
  speed_A-speed_B : Saturate  UpperLimit=speed_B  LowerLimit=speed_A
  wm^3 : Fcn  Expr=u(1)^3
  Torque_cmd : Outport
  wires:
  Product1/1 -> Sum3/1
  0-inf/1 -> Product1/2
  Sum2/1 -> 0-inf/1
  Constant/1 -> Sum2/1
  "Gain "/1 -> 0-power_C/1
  Idq_grid_conv/1 -> Looses/3(Idq_grid_conv)
  Idqr/1 -> Looses/4(Idqr)
  Idqs/1 -> Looses/2(Idqs)
  Sum4/1 -> "0-inf "/1  "Pelec_ref"
  wm^3/1 -> "Gain "/1
  "pu->pu "/1 -> wm^3/1
  Sum3/1 -> 0-1/1
  "pu->pu  "/1 -> Sum4/1
  0-1/1 -> "pu->pu  "/1
  wr/1 -> "pu->pu "/1, Sum2/2, speed_A-speed_B/1, Looses/1(wr), Switch/2, 1e-6-inf/1
  0-power_C/1 -> Switch/1
  Product3/1 -> Switch/3
  Constant1/1 -> Sum5/2
  speed_A-speed_B/1 -> Sum5/1
  Sum5/1 -> Product3/1
  Switch/1 -> Sum3/2
  Slope_D_C/1(Slope) -> Product1/1
  Slope_B_A/1(Slope) -> Product3/2
  "0-inf "/1 -> Product2/1
  1e-6-inf/1 -> Product2/2
  Product2/1 -> Torque_cmd/1
  Looses/1(P_looses) -> Sum4/2
  Freq/1 -> Looses/5(Freq)

== system SSN_39busRT_Ctrl_4WT_19B/SM_master/4 WT/SS_windfarm1to2/Wind Farm (DFIG Type)/Wind Turbine Doubly-Fed Induction Generator (Average Model)1/Control System_average/Control/Rotor-side converter Control system/Torque control/Torque regulator ==
  Torque_cmd : Inport
  Vdqs : Inport  Port=2
  Idqs : Inport  Port=3
  Freq : Inport  Port=4
  50%-inf : Saturate  UpperLimit=inf  LowerLimit=0.5
  Divide2 : Product  Inputs=*/
  Divide3 : Product  Inputs=**
  Lm/Ls : Constant  Value=Lm/(Lls+Lm)
  Rate Limiter : RateLimiter  RisingSlewLimit=current_slew_rate  FallingSlewLimit=-current_slew_rate
  Saturation : Saturate  UpperLimit=1  LowerLimit=0
  Stator flux estimator : Subsystem
  Idr : Outport
  wires:
  Saturation/1 -> Idr/1
  Rate Limiter/1 -> Saturation/1
  Freq/1 -> Stator flux estimator/3(Freq)
  Divide2/1 -> Rate Limiter/1
  Idqs/1 -> Stator flux estimator/2(Idqs)
  Torque_cmd/1 -> Divide2/1
  Vdqs/1 -> Stator flux estimator/1(Vdqs)
  Divide3/1 -> Divide2/2
  Stator flux estimator/1(Mag_Flux) -> 50%-inf/1
  50%-inf/1 -> Divide3/1
  Lm/Ls/1 -> Divide3/2

== system SSN_39busRT_Ctrl_4WT_19B/SM_master/4 WT/SS_windfarm1to2/Wind Farm (DFIG Type)1/Wind Turbine Doubly-Fed Induction Generator (Average Model)1/Control System_average/Control/Rotor-side converter Control system/Torque control/Torque reference ==
  wr : Inport
  Idqs : Inport  Port=2
  Idqr : Inport  Port=3
  Idq_grid_conv : Inport  Port=4
  Freq : Inport  Port=5
  0-1 : Saturate  UpperLimit=1  LowerLimit=0
  0-inf : Saturate  UpperLimit=inf  LowerLimit=0
  "0-inf " : Saturate  UpperLimit=inf  LowerLimit=0
  0-power_C : Saturate  UpperLimit=power_C  LowerLimit=0
  1e-6-inf : Saturate  UpperLimit=inf  LowerLimit=1e-6
  Constant : Constant  Value=speed_C
  Constant1 : Constant  Value=speed_A
  "Gain " : Gain  Gain=power_C  SaturateOnIntegerOverflow=on  OutDataTypeStr=Inherit: Same as input  ParamDataTypeStr=Inherit: Same as input
  Looses : Subsystem
  Product1 : Product  SaturateOnIntegerOverflow=on  OutDataTypeStr=Inherit: Same as first input
  Product2 : Product  Inputs=*/  SaturateOnIntegerOverflow=on  OutDataTypeStr=Inherit: Same as first input
  Product3 : Product  SaturateOnIntegerOverflow=on  OutDataTypeStr=Inherit: Same as first input
  Slope_B_A : Subsystem
  Slope_D_C : Subsystem
  Sum2 : Sum  Inputs=|-+  SaturateOnIntegerOverflow=on
  Sum3 : Sum  Inputs=|++  SaturateOnIntegerOverflow=on
  Sum4 : Sum  Inputs=|+-  SaturateOnIntegerOverflow=on
  Sum5 : Sum  Inputs=|+-  SaturateOnIntegerOverflow=on
  Switch : Switch  Threshold=speed_B  SaturateOnIntegerOverflow=on
  "pu->pu " : Gain  Gain=1/speed_C  SaturateOnIntegerOverflow=on  OutDataTypeStr=Inherit: Same as input  ParamDataTypeStr=Inherit: Same as input
  "pu->pu  " : Gain  Gain=Pmec/Pnom  SaturateOnIntegerOverflow=on  OutDataTypeStr=Inherit: Same as input  ParamDataTypeStr=Inherit: Same as input
  speed_A-speed_B : Saturate  UpperLimit=speed_B  LowerLimit=speed_A
  wm^3 : Fcn  Expr=u(1)^3
  Torque_cmd : Outport
  wires:
  Freq/1 -> Looses/5(Freq)
  Looses/1(P_looses) -> Sum4/2
  Product2/1 -> Torque_cmd/1
  1e-6-inf/1 -> Product2/2
  "0-inf "/1 -> Product2/1
  Slope_B_A/1(Slope) -> Product3/2
  Slope_D_C/1(Slope) -> Product1/1
  Switch/1 -> Sum3/2
  Sum5/1 -> Product3/1
  speed_A-speed_B/1 -> Sum5/1
  Constant1/1 -> Sum5/2
  Product3/1 -> Switch/3
  0-power_C/1 -> Switch/1
  wr/1 -> 1e-6-inf/1, Switch/2, Looses/1(wr), speed_A-speed_B/1, Sum2/2, "pu->pu "/1
  0-1/1 -> "pu->pu  "/1
  "pu->pu  "/1 -> Sum4/1
  Sum3/1 -> 0-1/1
  "pu->pu "/1 -> wm^3/1
  wm^3/1 -> "Gain "/1
  Sum4/1 -> "0-inf "/1  "Pelec_ref"
  Idqs/1 -> Looses/2(Idqs)
  Idqr/1 -> Looses/4(Idqr)
  Idq_grid_conv/1 -> Looses/3(Idq_grid_conv)
  "Gain "/1 -> 0-power_C/1
  Constant/1 -> Sum2/1
  Sum2/1 -> 0-inf/1
  0-inf/1 -> Product1/2
  Product1/1 -> Sum3/1

== system SSN_39busRT_Ctrl_4WT_19B/SM_master/4 WT/SS_windfarm1to2/Wind Farm (DFIG Type)1/Wind Turbine Doubly-Fed Induction Generator (Average Model)1/Control System_average/Control/Rotor-side converter Control system/Torque control/Torque regulator ==
  Torque_cmd : Inport
  Vdqs : Inport  Port=2
  Idqs : Inport  Port=3
  Freq : Inport  Port=4
  50%-inf : Saturate  UpperLimit=inf  LowerLimit=0.5
  Divide2 : Product  Inputs=*/
  Divide3 : Product  Inputs=**
  Lm/Ls : Constant  Value=Lm/(Lls+Lm)
  Rate Limiter : RateLimiter  RisingSlewLimit=current_slew_rate  FallingSlewLimit=-current_slew_rate
  Saturation : Saturate  UpperLimit=1  LowerLimit=0
  Stator flux estimator : Subsystem
  Idr : Outport
  wires:
  Lm/Ls/1 -> Divide3/2
  50%-inf/1 -> Divide3/1
  Stator flux estimator/1(Mag_Flux) -> 50%-inf/1
  Divide3/1 -> Divide2/2
  Vdqs/1 -> Stator flux estimator/1(Vdqs)
  Torque_cmd/1 -> Divide2/1
  Idqs/1 -> Stator flux estimator/2(Idqs)
  Divide2/1 -> Rate Limiter/1
  Freq/1 -> Stator flux estimator/3(Freq)
  Rate Limiter/1 -> Saturation/1
  Saturation/1 -> Idr/1

== system SSN_39busRT_Ctrl_4WT_19B/SM_master/4 WT/SS_windfarm3to4/Wind Farm (DFIG Type)/Wind Turbine Doubly-Fed Induction Generator (Average Model)1/Control System_average/Control/Rotor-side converter Control system/Torque control/Torque reference ==
  wr : Inport
  Idqs : Inport  Port=2
  Idqr : Inport  Port=3
  Idq_grid_conv : Inport  Port=4
  Freq : Inport  Port=5
  0-1 : Saturate  UpperLimit=1  LowerLimit=0
  0-inf : Saturate  UpperLimit=inf  LowerLimit=0
  "0-inf " : Saturate  UpperLimit=inf  LowerLimit=0
  0-power_C : Saturate  UpperLimit=power_C  LowerLimit=0
  1e-6-inf : Saturate  UpperLimit=inf  LowerLimit=1e-6
  Constant : Constant  Value=speed_C
  Constant1 : Constant  Value=speed_A
  "Gain " : Gain  Gain=power_C  SaturateOnIntegerOverflow=on  OutDataTypeStr=Inherit: Same as input  ParamDataTypeStr=Inherit: Same as input
  Looses : Subsystem
  Product1 : Product  SaturateOnIntegerOverflow=on  OutDataTypeStr=Inherit: Same as first input
  Product2 : Product  Inputs=*/  SaturateOnIntegerOverflow=on  OutDataTypeStr=Inherit: Same as first input
  Product3 : Product  SaturateOnIntegerOverflow=on  OutDataTypeStr=Inherit: Same as first input
  Slope_B_A : Subsystem
  Slope_D_C : Subsystem
  Sum2 : Sum  Inputs=|-+  SaturateOnIntegerOverflow=on
  Sum3 : Sum  Inputs=|++  SaturateOnIntegerOverflow=on
  Sum4 : Sum  Inputs=|+-  SaturateOnIntegerOverflow=on
  Sum5 : Sum  Inputs=|+-  SaturateOnIntegerOverflow=on
  Switch : Switch  Threshold=speed_B  SaturateOnIntegerOverflow=on
  "pu->pu " : Gain  Gain=1/speed_C  SaturateOnIntegerOverflow=on  OutDataTypeStr=Inherit: Same as input  ParamDataTypeStr=Inherit: Same as input
  "pu->pu  " : Gain  Gain=Pmec/Pnom  SaturateOnIntegerOverflow=on  OutDataTypeStr=Inherit: Same as input  ParamDataTypeStr=Inherit: Same as input
  speed_A-speed_B : Saturate  UpperLimit=speed_B  LowerLimit=speed_A
  wm^3 : Fcn  Expr=u(1)^3
  Torque_cmd : Outport
  wires:
  Product1/1 -> Sum3/1
  0-inf/1 -> Product1/2
  Sum2/1 -> 0-inf/1
  Constant/1 -> Sum2/1
  "Gain "/1 -> 0-power_C/1
  Idq_grid_conv/1 -> Looses/3(Idq_grid_conv)
  Idqr/1 -> Looses/4(Idqr)
  Idqs/1 -> Looses/2(Idqs)
  Sum4/1 -> "0-inf "/1  "Pelec_ref"
  wm^3/1 -> "Gain "/1
  "pu->pu "/1 -> wm^3/1
  Sum3/1 -> 0-1/1
  "pu->pu  "/1 -> Sum4/1
  0-1/1 -> "pu->pu  "/1
  wr/1 -> "pu->pu "/1, Sum2/2, speed_A-speed_B/1, Looses/1(wr), Switch/2, 1e-6-inf/1
  0-power_C/1 -> Switch/1
  Product3/1 -> Switch/3
  Constant1/1 -> Sum5/2
  speed_A-speed_B/1 -> Sum5/1
  Sum5/1 -> Product3/1
  Switch/1 -> Sum3/2
  Slope_D_C/1(Slope) -> Product1/1
  Slope_B_A/1(Slope) -> Product3/2
  "0-inf "/1 -> Product2/1
  1e-6-inf/1 -> Product2/2
  Product2/1 -> Torque_cmd/1
  Looses/1(P_looses) -> Sum4/2
  Freq/1 -> Looses/5(Freq)

== system SSN_39busRT_Ctrl_4WT_19B/SM_master/4 WT/SS_windfarm3to4/Wind Farm (DFIG Type)/Wind Turbine Doubly-Fed Induction Generator (Average Model)1/Control System_average/Control/Rotor-side converter Control system/Torque control/Torque regulator ==
  Torque_cmd : Inport
  Vdqs : Inport  Port=2
  Idqs : Inport  Port=3
  Freq : Inport  Port=4
  50%-inf : Saturate  UpperLimit=inf  LowerLimit=0.5
  Divide2 : Product  Inputs=*/
  Divide3 : Product  Inputs=**
  Lm/Ls : Constant  Value=Lm/(Lls+Lm)
  Rate Limiter : RateLimiter  RisingSlewLimit=current_slew_rate  FallingSlewLimit=-current_slew_rate
  Saturation : Saturate  UpperLimit=1  LowerLimit=0
  Stator flux estimator : Subsystem
  Idr : Outport
  wires:
  Saturation/1 -> Idr/1
  Rate Limiter/1 -> Saturation/1
  Freq/1 -> Stator flux estimator/3(Freq)
  Divide2/1 -> Rate Limiter/1
  Idqs/1 -> Stator flux estimator/2(Idqs)
  Torque_cmd/1 -> Divide2/1
  Vdqs/1 -> Stator flux estimator/1(Vdqs)
  Divide3/1 -> Divide2/2
  Stator flux estimator/1(Mag_Flux) -> 50%-inf/1
  50%-inf/1 -> Divide3/1
  Lm/Ls/1 -> Divide3/2

== system SSN_39busRT_Ctrl_4WT_19B/SM_master/4 WT/SS_windfarm3to4/Wind Farm (DFIG Type)2/Wind Turbine Doubly-Fed Induction Generator (Average Model)1/Control System_average/Control/Rotor-side converter Control system/Torque control/Torque reference ==
  wr : Inport
  Idqs : Inport  Port=2
  Idqr : Inport  Port=3
  Idq_grid_conv : Inport  Port=4
  Freq : Inport  Port=5
  0-1 : Saturate  UpperLimit=1  LowerLimit=0
  0-inf : Saturate  UpperLimit=inf  LowerLimit=0
  "0-inf " : Saturate  UpperLimit=inf  LowerLimit=0
  0-power_C : Saturate  UpperLimit=power_C  LowerLimit=0
  1e-6-inf : Saturate  UpperLimit=inf  LowerLimit=1e-6
  Constant : Constant  Value=speed_C
  Constant1 : Constant  Value=speed_A
  "Gain " : Gain  Gain=power_C  SaturateOnIntegerOverflow=on  OutDataTypeStr=Inherit: Same as input  ParamDataTypeStr=Inherit: Same as input
  Looses : Subsystem
  Product1 : Product  SaturateOnIntegerOverflow=on  OutDataTypeStr=Inherit: Same as first input
  Product2 : Product  Inputs=*/  SaturateOnIntegerOverflow=on  OutDataTypeStr=Inherit: Same as first input
  Product3 : Product  SaturateOnIntegerOverflow=on  OutDataTypeStr=Inherit: Same as first input
  Slope_B_A : Subsystem
  Slope_D_C : Subsystem
  Sum2 : Sum  Inputs=|-+  SaturateOnIntegerOverflow=on
  Sum3 : Sum  Inputs=|++  SaturateOnIntegerOverflow=on
  Sum4 : Sum  Inputs=|+-  SaturateOnIntegerOverflow=on
  Sum5 : Sum  Inputs=|+-  SaturateOnIntegerOverflow=on
  Switch : Switch  Threshold=speed_B  SaturateOnIntegerOverflow=on
  "pu->pu " : Gain  Gain=1/speed_C  SaturateOnIntegerOverflow=on  OutDataTypeStr=Inherit: Same as input  ParamDataTypeStr=Inherit: Same as input
  "pu->pu  " : Gain  Gain=Pmec/Pnom  SaturateOnIntegerOverflow=on  OutDataTypeStr=Inherit: Same as input  ParamDataTypeStr=Inherit: Same as input
  speed_A-speed_B : Saturate  UpperLimit=speed_B  LowerLimit=speed_A
  wm^3 : Fcn  Expr=u(1)^3
  Torque_cmd : Outport
  wires:
  Freq/1 -> Looses/5(Freq)
  Looses/1(P_looses) -> Sum4/2
  Product2/1 -> Torque_cmd/1
  1e-6-inf/1 -> Product2/2
  "0-inf "/1 -> Product2/1
  Slope_B_A/1(Slope) -> Product3/2
  Slope_D_C/1(Slope) -> Product1/1
  Switch/1 -> Sum3/2
  Sum5/1 -> Product3/1
  speed_A-speed_B/1 -> Sum5/1
  Constant1/1 -> Sum5/2
  Product3/1 -> Switch/3
  0-power_C/1 -> Switch/1
  wr/1 -> 1e-6-inf/1, Switch/2, Looses/1(wr), speed_A-speed_B/1, Sum2/2, "pu->pu "/1
  0-1/1 -> "pu->pu  "/1
  "pu->pu  "/1 -> Sum4/1
  Sum3/1 -> 0-1/1
  "pu->pu "/1 -> wm^3/1
  wm^3/1 -> "Gain "/1
  Sum4/1 -> "0-inf "/1  "Pelec_ref"
  Idqs/1 -> Looses/2(Idqs)
  Idqr/1 -> Looses/4(Idqr)
  Idq_grid_conv/1 -> Looses/3(Idq_grid_conv)
  "Gain "/1 -> 0-power_C/1
  Constant/1 -> Sum2/1
  Sum2/1 -> 0-inf/1
  0-inf/1 -> Product1/2
  Product1/1 -> Sum3/1

== system SSN_39busRT_Ctrl_4WT_19B/SM_master/4 WT/SS_windfarm3to4/Wind Farm (DFIG Type)2/Wind Turbine Doubly-Fed Induction Generator (Average Model)1/Control System_average/Control/Rotor-side converter Control system/Torque control/Torque regulator ==
  Torque_cmd : Inport
  Vdqs : Inport  Port=2
  Idqs : Inport  Port=3
  Freq : Inport  Port=4
  50%-inf : Saturate  UpperLimit=inf  LowerLimit=0.5
  Divide2 : Product  Inputs=*/
  Divide3 : Product  Inputs=**
  Lm/Ls : Constant  Value=Lm/(Lls+Lm)
  Rate Limiter : RateLimiter  RisingSlewLimit=current_slew_rate  FallingSlewLimit=-current_slew_rate
  Saturation : Saturate  UpperLimit=1  LowerLimit=0
  Stator flux estimator : Subsystem
  Idr : Outport
  wires:
  Lm/Ls/1 -> Divide3/2
  50%-inf/1 -> Divide3/1
  Stator flux estimator/1(Mag_Flux) -> 50%-inf/1
  Divide3/1 -> Divide2/2
  Vdqs/1 -> Stator flux estimator/1(Vdqs)
  Torque_cmd/1 -> Divide2/1
  Idqs/1 -> Stator flux estimator/2(Idqs)
  Divide2/1 -> Rate Limiter/1
  Freq/1 -> Stator flux estimator/3(Freq)
  Rate Limiter/1 -> Saturation/1
  Saturation/1 -> Idr/1
